simulink model "wlan_phy_tx_pmd"  (Simulink 7.8)
settings: Solver=VariableStepDiscrete  SolverMode=SingleTasking  StartTime=0.0  StopTime=inf  RelTol=1e-3
PostLoadFcn:
  | wlan_phy_tx_init
InitFcn:
  | wlan_phy_tx_init
StartFcn:
  | wlan_phy_tx_init
undefined symbols (not defined in the file): gcbh, ht_preamble_rom, MAX_CP_LEN, MAX_DATA_BITS_PER_SYM_PERIOD, MAX_NCBPS, MAX_NUM_BYTES, MAX_NUM_SC, MAX_NUM_SYMS, mcs_rom_11ag, mcs_rom_11n, Mod_Constellation_16QAM, Mod_Constellation_64QAM, Mod_Constellation_BPSK, Mod_Constellation_QPSK, Preamble_IQ, Preamble_IQ_scaled, tx_sim, wlan_tx_interleave_rom, xlBlockLoadCallback, xlGetNormalizedPeriod
libraries: xbsIndex_r4 x1358, xbsEDKLib_r4 x1
(part 1 of 10)
settings Model: Creator=murphpo  LastModifiedBy=murphpo
settings OptimizationCC: InlineParams=on
settings DebuggingCC: SolverPrmCheckMsg=none  UnconnectedInputMsg=none  UnconnectedOutputMsg=none  UnconnectedLineMsg=none

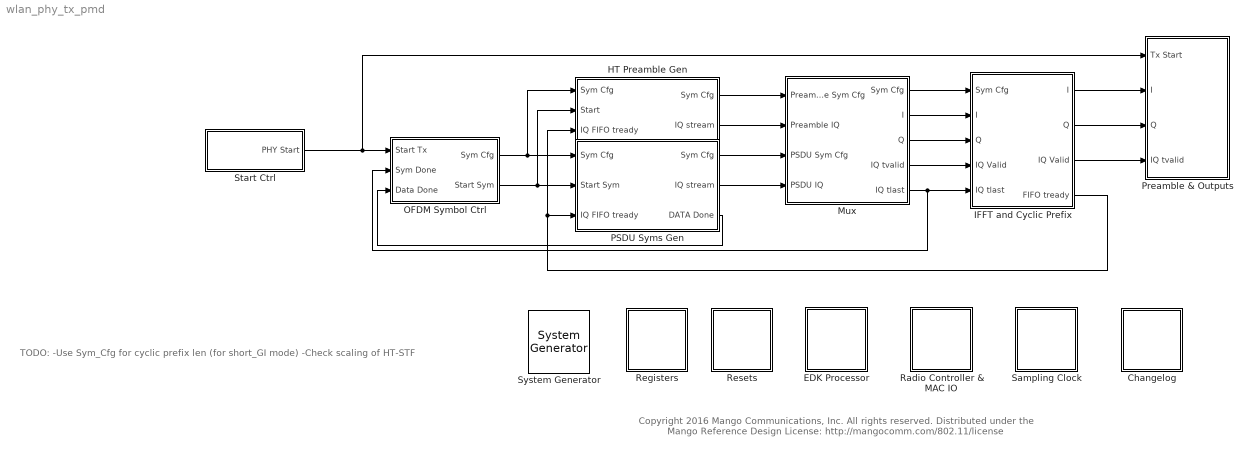
== system wlan_phy_tx_pmd ==
  note: Copyright 2016 Mango Communications, Inc. All rights reserved.
      |
      | Distributed under the Mango Reference Design License:
      | http://mangocomm.com/802.11/license
  note: TODO:
      | -Use Sym_Cfg for cyclic prefix len (for short_GI mode)
      | -Check scaling of HT-STF
  " System Generator" : xbsIndex_r4/ System Generator  Tag=genX  xilinxfamily=virtex6  part=xc6vlx240t  speed=-2  package=ff1156  synthesis_tool=XST  clock_wrapper=Clock Enables  directory=./pcore_tx_v414  proj_type=Project Navigator  Synth_file=XST Defaults  Impl_file=ISE Defaults  testbench=off  simulink_period=1  sysclk_period=6.25  dcm_input_clock_period=10  incr_netlist=off  trim_vbits=Everywhere in SubSystem  dbl_ovrd=According to Block Masks  core_generation=According to Block Masks  run_coregen=off  deprecated_control=off  eval_field=0  block_type=sysgen
  Changelog : Subsystem
  EDK Processor : Subsystem  LoadFcn=xlBlockLoadCallback(gcbh);  mask(Xilinx EDK Processor Block){mode=EDK pcore generation, xmp=, MemVisToProc=<qt bgcolor="#FFFFFF"><div><img src="S:/Xilinx/14.4/ISE_DS/ISE/sysgen/data/images/registerplus.gif"> &lt;&lt;Timing&gt;&gt;<br></div><div><img src="S:/Xilinx/14.4/ISE_DS/ISE/sysgen/data/images/registerplus.gif"> &lt;&lt;Config&gt;&gt;<br></div><div><img src="S:/Xilinx/14.4/ISE_DS/ISE/sysgen/data/images/registerplus.gif"> &lt;&lt;PKT_BUF_SEL&gt;&gt;<br></div><div><img src="S:/Xilinx/14.4/ISE_DS/ISE/sysgen/data/images/registerplus.gif"> &lt;&lt;Output_Scaling&gt;&gt;<br></div><div><img src="S:/Xilinx/14.4/ISE_DS/ISE/sysgen/data/images/registerplus.gif"> &lt;&lt;TX_START&gt;&gt;<br></div><div><img src="S:/Xilinx/14.4/ISE_DS/ISE/sysgen/data/images/registerplus.gif"> &lt;&lt;FFT_Config&gt;&gt;<br></div><div><img src="S:/Xilinx/14.4/ISE_DS/ISE/sysgen/data/images/registerplus.gif"> &lt;&lt;STATUS&gt;&gt;<br></div></qt>, AvailableMemories=<empty>, portInterfaceTable={'exposed'=>[],'portdir'=>[],'portname'=>[],'shortname'=>[]}, bus_type_sgadvanced=, bus_type=AXI, baseaddr=0x80000000, baseaddr_lock_sgadvanced=, baseaddr_lock=off, dual_clock_sgadvanced=, dual_clock=on, reg_readback_sgadvanced=, reg_readback=on, ucf_file=, inheritDeviceType_sgadvanced=, inheritDeviceType=off, elf_file=, codebug_sgadvanced=, codebug=on, clock_name=plb, internalPortList={}, resetPolarity=0, memxtable={'mladdr'=>[0.00000000000000000,1.00000000000000000,2.00000000000000000,3.00000000000000000,4.00000000000000000,5.00000000000000000,0.00000000000000000],'mlist'=>['wlan_phy_tx_pmd/Registers/From Register6','wlan_phy_tx_pmd/Registers/From Register5','wlan_phy_tx_pmd/Registers/From Register4','wlan_phy_tx_pmd/Registers/From Register3','wlan_phy_tx_pmd/Registers/From Register2','wlan_phy_tx_pmd/Registers/From Register1','wlan_phy_tx_pmd/Registers/To Register'],'mlname'=>['\\'Timing\\'','\\'Config\\'','\\'PKT_BUF_SEL\\'','\\'Output_Scaling\\'','\\'TX_START\\'','\\'FFT_Config\\'','\\'STATUS\\''],'mlstate'=>[0.00000000000000000,0.00000000000000000,0.00000000000000000,0.00000000000000000,0.00000000000000000,0.00000000000000000,0.00000000000000000]}, procinfo={}, memmapdirty=off, blockname=, xpsintstyle=default, has_advanced_control=0, sggui_pos=-1,-1,-1,-1, block_type=edkprocessor, block_version=2.7, sg_icon_stat=58,60,-1,-1,white,blue,0,07734,right,,[ ],[ ], sg_mask_display=|, sg_list_contents={'table'=>{'AvailableMemories'=>'popup(<empty>)'}}, sg_blockgui_xml=}
      mask sg_mask_display=|
      | fprintf('','COMMENT: begin icon graphics');
      | patch([0 58 58 0 0 ],[0 0 60 60 0 ],[0.77 0.82 0.91 ]);
      | plot([0 58 58 0 0 ],[0 0 60 60 0 ]);
      | patch([11.2 22.76 30.76 38.76 46.76 30.76 19.2 11.2 ],[38.88 38.88 46.88 38.88 46.88 46.88 46.88 38.88 ],[1 1 1 ]);
      | patch([19.2 30.76 22.76 11.2 19.2 ],[30.88 30.88 38.88 38.88 30.88 ],[0.931 0.946 0.973 ]);
      | patch([11.2 22.76 30.76 19.2 11.2 ],[22.88 22.88 30.88 30.88 22.88 ],[1 1 1 ]);
      | patch([19.2 46.76 38.76 30.76 22.76 11.2 19.2 ],[14.88 14.88 22.88 14.88 22.88 22.88 14.88 ],[0.931 0.946 0.973 ]);
      | fprintf('','COMMENT: end icon graphics');
      | fprintf('','COMMENT: begin icon text');
      | fprintf('','COMMENT: end icon text');
      mask prompts: mode "Configure Processor for"; xmp "XPS Project"; MemVisToProc ""; AvailableMemories "Available Memories"; portInterfaceTable ""; bus_type_sgadvanced ""; bus_type "Bus Type"; baseaddr "Base Address"; baseaddr_lock_sgadvanced ""; baseaddr_lock "Lock"; dual_clock_sgadvanced ""; dual_clock "Dual Clocks"; reg_readback_sgadvanced ""; reg_readback "Register Read-Back"; ucf_file "Constraint File"; inheritDeviceType_sgadvanced ""; inheritDeviceType "Inherit Device Type"; elf_file "Initial Program"; codebug_sgadvanced ""; codebug "Enable Co-Debug with Xilinx SDK (Beta)"; clock_name ""; internalPortList ""; resetPolarity ""; memxtable ""; procinfo ""; memmapdirty ""; blockname ""; xpsintstyle ""; has_advanced_control ""; sggui_pos ""; block_type ""; block_version ""; sg_icon_stat ""; sg_mask_display ""; sg_list_contents ""; sg_blockgui_xml ""
      mask help: Xilinx EDK Processor
      mask init:
      | try
      |   tmp_gcb = gcb;
      |   tmp_gcbh = gcbh;
      |   if (strcmp('SysGenIndex',get_param(bdroot(tmp_gcbh),'tag')) && ~isempty(regexp(bdroot(tmp_gcb), '^xbs', 'once')))
      |     return;
      |   end;
      |   xlMungeMaskParams;
      | 
      |   block_type='edkprocessor';
      | 
      |   serialized_declarations = '{''block_type''=>''String''}';
      |   xledkprocessor_init();
      |   ptable_ = xlblockprep(get_param(tmp_gcb, 'MaskWSVariables'));
      |   try
      |     xlBlockMoveCallback(tmp_gcbh);
      |   catch 
      |      clear global xl_updateicon_recursion_guard;
      |   end;
      | catch
      |   global dbgsysgen;
      |   if(~isempty(dbgsysgen) && dbgsysgen)
      |     e = regexprep(lasterr, '\n', '\nError: ');
      |     disp(['Error: While running MaskInit code on block ' tmp_gcb ': ' e]);
      |     error(e);
      |   end
      | end
      settings: CopyFcn=xlProcBlockCopyCallback(gcbh);xlBlockMoveCallback(gcbh);  DeleteFcn=xlDestroyGui(gcbh);  ModelCloseFcn=xlDestroyGui(gcbh);  PreSaveFcn=xlBlockPreSaveCallback(gcbh);  PostSaveFcn=xlBlockPostSaveCallback(gcbh);  DestroyFcn=xlDestroyGui(gcbh);  OpenFcn=bh=gcbh;xlProcBlockCallbacks('populatesharedmemorylistbox',bh);xlOpenGui(bh, 'edkprocessor_gui.xml', @xlProcBlockEnablement, @xlProcBlockAction);  CloseFcn=xlDestroyGui(gcbh);  MoveFcn=xlBlockMoveCallback(gcbh);
      mask Help: eval('');xlDoc('-book','sysgen','-topic','EDK_Processor');
      mask StyleString: popup(EDK pcore generation|HDL netlisting),edit,edit,edit,edit,edit,popup(AXI|PLB),edit,edit,checkbox,edit,checkbox,edit,checkbox,edit,edit,checkbox,edit,edit,checkbox,edit,edit,edit,edit,edit,edit,edit,edit,edit,edit,edit,edit,edit,edit,edit,edit
      mask Display:
      | fprintf('','COMMENT: begin icon graphics');
      | patch([0 58 58 0 0 ],[0 0 60 60 0 ],[0.77 0.82 0.91 ]);
      | plot([0 58 58 0 0 ],[0 0 60 60 0 ]);
      | patch([11.2 22.76 30.76 38.76 46.76 30.76 19.2 11.2 ],[38.88 38.88 46.88 38.88 46.88 46.88 46.88 38.88 ],[1 1 1 ]);
      | patch([19.2 30.76 22.76 11.2 19.2 ],[30.88 30.88 38.88 38.88 30.88 ],[0.931 0.946 0.973 ]);
      | patch([11.2 22.76 30.76 19.2 11.2 ],[22.88 22.88 30.88 30.88 22.88 ],[1 1 1 ]);
      | patch([19.2 46.76 38.76 30.76 22.76 11.2 19.2 ],[14.88 14.88 22.88 14.88 22.88 22.88 14.88 ],[0.931 0.946 0.973 ]);
      | fprintf('','COMMENT: end icon graphics');
      | fprintf('','COMMENT: begin icon text');
      | fprintf('','COMMENT: end icon text');
  HT Preamble Gen : Subsystem
  IFFT and Cyclic Prefix : Subsystem
  Mux : Subsystem
  OFDM Symbol Ctrl : Subsystem
  PSDU Syms Gen : Subsystem
  Preamble & Outputs : Subsystem
  Radio Controller & MAC IO : Subsystem
  Registers : Subsystem
  Resets : Subsystem
  Sampling Clock : Subsystem
  Start Ctrl : Subsystem
  wires:
  IFFT and Cyclic Prefix/1(" I") -> Preamble & Outputs/2(I)
  IFFT and Cyclic Prefix/2(" Q") -> Preamble & Outputs/3(Q)
  IFFT and Cyclic Prefix/3(" IQ Valid") -> Preamble & Outputs/4(IQ tvalid)
  Mux/5(IQ tlast) -> OFDM Symbol Ctrl/2(Sym Done), IFFT and Cyclic Prefix/5(IQ tlast)
  HT Preamble Gen/1(" Sym Cfg") -> Mux/1(Preamble Sym Cfg)
  HT Preamble Gen/2(IQ stream) -> Mux/2(Preamble IQ)
  PSDU Syms Gen/1(" Sym Cfg") -> Mux/3(PSDU Sym Cfg)
  PSDU Syms Gen/2(IQ stream) -> Mux/4(PSDU IQ)
  OFDM Symbol Ctrl/1(Sym Cfg) -> PSDU Syms Gen/1(Sym Cfg), HT Preamble Gen/1(Sym Cfg)
  OFDM Symbol Ctrl/2(" Start Sym") -> PSDU Syms Gen/2(Start Sym), HT Preamble Gen/2(Start)
  Start Ctrl/1(PHY Start) -> OFDM Symbol Ctrl/1(Start Tx), Preamble & Outputs/1(Tx Start)
  IFFT and Cyclic Prefix/4(FIFO tready) -> HT Preamble Gen/3(IQ FIFO tready), PSDU Syms Gen/3(IQ FIFO tready)
  Mux/1(Sym Cfg) -> IFFT and Cyclic Prefix/1(Sym Cfg)
  Mux/2(" I") -> IFFT and Cyclic Prefix/2(I)
  Mux/3(" Q") -> IFFT and Cyclic Prefix/3(Q)
  Mux/4(" IQ tvalid") -> IFFT and Cyclic Prefix/4(IQ Valid)
  PSDU Syms Gen/3(DATA Done) -> OFDM Symbol Ctrl/3(Data Done)

== system wlan_phy_tx_pmd/Changelog ==
  note: 2.00.a:
      | -First export as _pmd, with I/O for mac_hw integration
      |
      | 2.00.b:
      | -Changed pkt buf interface to 64b
      | -Added pkt buf addr offset
      |
      | 2.00.c:
      | -Fixed puncturing timing
      | -Enabled BPSK/QPSK 3/4 schemes
      |
      | 2.00.d:
      | -Attempting fix of bad pkt Tx (based on wireshark Rx checksum)
      |   at 3/4; suspected bug in not puncturing TAIL
      |
      | 2.00.e:
      | -Reworked TxEn disable logic with programmable extension
      |   -Moved TX_END extension to new register
      |
      | 2.00.f:
      | -Added longer Tx -> Rx delay (250 cycles) to reduce RSSI/ADC
      |   transients at Rx post Tx
      |
      | 2.00.g:
      | -Added RX_SIGS_INVALID output to supress post-Tx transients from
      |   ADCs at input to PHY Rx
      |
      | 2.00.h:
      | -Added 16QAM support
      |   -64QAM is trickier; interleaver will need new arch, since 1->6 isn't a supported DPRAM aspect ratio
      |
      | 2.00.i:
      | -Added 64QAM support
      |
      | 2.00.j:
      | -Fixed slip-by-1-per-symbol bug in FFT start timing (broke long-duration pkts)
      | -Added reg bit to not reset scrambling LFSR per pkt
      |
      | 2.00.k:
      | -Added RF B DAC outputs; A/B selection done via config register
      |
      | 2.00.l:
      | -Fixed zero sample between preamble and first OFDM symbol
      | -Removed unused reset port
      |
      | 2.00.m:
      | -More output mux timing bug fixes (last sample of pkt was being dropped)
      |
      | 2.00.n:
      | -Added explicit DAC_TX_CLK input to replace upsampled T=8 constant as IQ clock enable
      | -Replaced delays with registers in preamble output delays
      | -Added (x || FORCE_RESET) to SR latches in start ctrl (trying to fix very rare perma-Tx mode on download)
      | -Added (x || posedge(tx_start)) to output FIFO reset (trying to fix very rare extra sample between LTS - SIGNAL)
      |
      | -2.00.o:
      | -Added RFC,D outputs
      |
      | 2.00.p:
      | -More pipeline registers throughput (sw regs and outputs mostly)
      |
      | 2.00.q:
      | -Added logic to insert MAC timestamp in outgoing packets. Timestamp is 8 bytes. Start/stop byte
      |   indexes are set by sw. Timestamp must start on 8-byte boundary (true for standard beacon/probe frames)
      |
      | 2.00.r:
      | -Added passthrough for Tx gain setting. Now MAC provides TxGain with each Tx (same as pkt buf sel). PHY
      |   passes this through to the radio controller user TxGain port.
      |
      | 2.00.s:
      | -Added Tx Ant Mask passthrough for MAC selection of active Tx antennas
      | -Added ctrl bits for:
      |   -En/disable use of MAC ant mask
      |   -Endian swap MAC ant mask before output to RC (will be removed when correct endianess is determined in hw)
      |
      | 2.00.t:
      | -Made SIGNAL.LENGTH max value programmable, in units of kB
      |
      | 2.00.u - 2.00.w:
      | -Added separate TX_GAIN paths per RF (MAC -> PHY -> radio_controller passthrough)
      | -Added delayed TX_RUNNING signal, to trigger pkt det at other nodes
      |
      | 2.00.x:
      | -Merged TX_RUNNING outputs (delayed, not-delayed) with mux to select
  note: 2.01.a:
      | -Cleaed up init script - no PHY design changes
      |
      | 2.01.b:
      | -Added pipeline regs between pkt buf and muxes
      |
      | 2.01.c:
      | -Fixed scaling of preamble/constellations to fix bad
      |   scaling of outer points for 64-QAM. New scaling will
      |   reduce effective Tx power 0.3dB; increase Tx_Scaling
      |   register value to compensate.
      | -Updated values for pilot tones to use BSPK constellation
      |   definition in init script (+/-1 were hard coded previously)
      |
      | 2.01.d:
      | -Replaced upsampled-constants with TX_IQ_SAMP_CE from
      |   in both start/add extension subsystems
  note: 4.00.a:
      | -Re-designed most of the Tx PHY pipeline
      |   -Added 11n SISO support
      |   -Replaced interleaver-per-mod with unified bits-in, syms-out interleaver
      |   -Replaced control logic with simpler generate-one-sym-at-a-time logic
      |   -Replcaed packet buffer addressing logic with simpler packet section slicing
      |   -Adopted external sample clock enable, now supports 5/10/20/40 MSps modes
      |   -Unified configuration params for each OFDM symbol in one subsystem
      |
      | -Added DFFs around output FIFO control signals, hoping to isolate apparent
      |   asychronous assertions
      | -Qualified PHY_Start by samp_ce, for fixed phase relationship between
      |   sample clock and PHY-MAC control
      |
      | 4.00.b:
      | -Fixed missing posedge on software RC_RXEN
      |
      | 4.00.c-e:
      | -Debugging missing interleaver RAM netlist
      | -Increased post-tx extension values to 10 bits
      |
      | 4.00.f:
      | -Added ping/pong interleaver RAMs, now supports 40MSps at all MCS
      |
      | 4.00.g:
      | -Fixed enable generation logic for output registers (was asserting late, truncating
      |   STS portion of preamble)
      |
      | 4.00.h:
      | -Fixed 11n pilot shifting sequence
  note: 2XCLK Branch - since merged
      |
      | 3.00.a:
      | Updated sim-only clock-enable gen to 4x
      |
      | 3.00.b:
      | Used local clk en gen (upsampled constant 4)
      |
      | 3.00.c:
      | Added ILA
      |
      | 3.00.d:
      | Removed ILA (debugging Rx)
      | Added DFF to DATA_IN, WREN, RST inputs of DAC FIFO, testing
      |   theory that an async write or reset is responsible for hw mismatch
      | NOTE: DFFs on FIFO inputs didn't resolve extra post-preamble sample. Observed
      |   good and bad Tx on multiple downloads of same design with 3.00.d Tx PHY.
      |
      | 3.00.e:
      | Qualified RC_PHY_TX_START by SAMP_CE (safe, since RC holds its outputs
      |   high until reset at end of Tx)
      | NOTE: didn't resolve issue; still see good/bad Tx on reconfig
      |
      | 3.00.f:
      | Added DFF to SAMP_CE before consumers in outputs block - testing theory that FIFO.RD
      |  somehow reacts one cycle late when generated by combinational logic
      | Re-enabled CS ILA
      |
      | 3.00.g:
      | Replaced upsampled constant with samp_ce gateway in
      | (this version has not exhibited any bad-Tx behavior in harware, yet)
      |
      | 3.00.h:
      | Disregarded ILA
      | Increased size of post-Tx timing values to 10 bits each (from 8)
